simulink model "Old_control_speed"  (R2023b)
settings: Solver=ode1  StartTime=0.0  StopTime=inf  FixedStep=0.01  RelTol=1e-3
libraries: qbmove_library x3, simulink x2, QB_pacer_lib x1
settings Model: Creator=ilari  LastModifiedBy=ilari

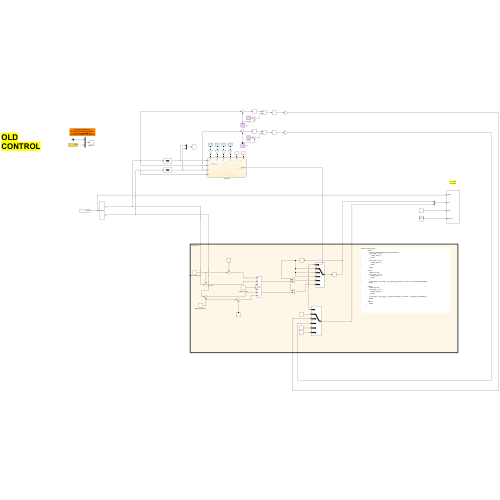
[thumbnail: Simulink's stored preview of the top-level diagram]
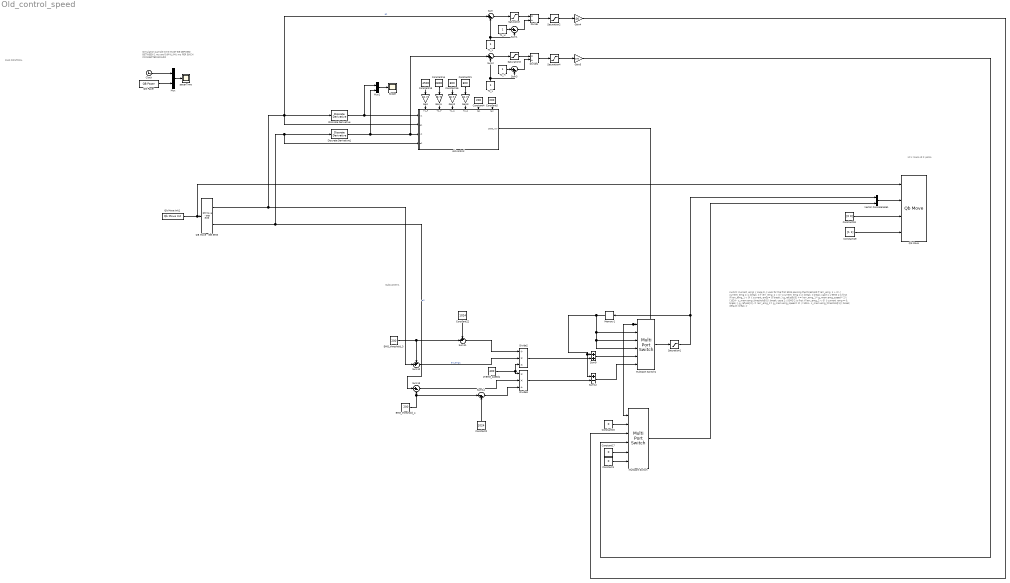
== system Old_control_speed ==
  note: Subsystem1
  note: OLD CONTROL
  note: id 1: mano
      | id 2: polso
  note: switch (current_emg) {
      | case 0:
      | // Look for the first EMG passing the threshold
      | if (err_emg_1 > 0) {
      | current_emg = 1;
      | break;
      | }
      | if (err_emg_2 > 0) {
      | current_emg = 2;
      | break;
      | }
      | break;
      |
      | case 1:
      | // EMG 1 is first
      | if (err_emg_1 < 0) {
      | current_emg = 0;
      | break;
      | }
      | g_ref.pos[0] += (err_emg_1 * g_mem.emg_speed * 2) / (1024 - c_mem.emg_threshold[0]);
      | break;
      |
      | case 2:
      | // EMG 2 is first
      | if (err_emg_2 < 0) {
      | current_emg = 0;
      | break;
      | }
      | g_ref.pos[0] -= (err_emg_2 * g_mem.emg_speed * 2) / (1024 - c_mem.emg_threshold[1]);
      | break;
      |
      | default:
      | break;
      | }
  note: Simulation sample time
      | MUST BE DEFINED BETWEEN
      | 1 ms and 0.6*N_IMU ms
      | PER EACH CONNECTED BOARD
  2*EMG_speed1 : Constant  Value=400
  Clock : Clock
  Constant1 : Constant  Value=0
  Constant13 : Constant  Value=4500
  Constant14 : Constant  Value=2800
  Constant15 : Constant  Value=0
  Constant16 : Constant  Value=800
  Constant17 : Constant  Value=0
  Constant18 : Constant  Value=[0 0]
  Constant19 : Constant  Value=[1 1]
  Constant2 : Constant  Value=1024
  Constant21 : Constant  Value=800
  Constant22 : Constant  Value=1024
  Constant4 : Constant  Value=200
  Constant5 : Constant  Value=200
  Discrete Derivative : simulink/Discrete/Discrete Derivative  gainval=1.0  ICPrevScaledInput=0.0  OutMin=[]  OutMax=[]  OutDataType=fixdt(1, 16)  OutScaling=2^-10  DoSatur=off
  Discrete Derivative1 : simulink/Discrete/Discrete Derivative  gainval=1.0  ICPrevScaledInput=0.0  OutMin=[]  OutMax=[]  OutDataType=fixdt(1, 16)  OutScaling=2^-10  DoSatur=off
  Divide : Product  Inputs=*/
  Divide1 : Product  Inputs=*/
  Divide2 : Product  Inputs=/**
  Divide3 : Product  Inputs=**/
  EMG_threshold_3 : Constant  Value=200
  EMG_threshold_4 : Constant  Value=200
  Gain{,1..3} (4 alike) : Gain  Gain=0.7
  Gain4 : Gain  Gain=100
  Gain5 : Gain  Gain=-100
  Memory1 : Memory
  Multiport Switch : MultiPortSwitch  DataPortOrder=Zero-based contiguous  Inputs=5  zeroidx=on  SaturateOnIntegerOverflow=off  InputSameDT=off
  Multiport Switch1 : MultiPortSwitch  DataPortOrder=Zero-based contiguous  Inputs=5  zeroidx=on  SaturateOnIntegerOverflow=off  InputSameDT=off
  Mux : Mux  Inputs=2
  Mux1 : Mux  Inputs=2
  QB Move - Get EMG : qbmove_library/QB Move - Get EMG  ID=2  DAISY_CHAINING=off
      settings: SourceProductName=Qb Move Library
  QB Pacer : QB_pacer_lib/QB Pacer  simTimePerRealTime=1
      settings: SourceProductName=QB Pacer
  Qb Move : qbmove_library/Qb Move  ID=[1 2]  ACTIVE_COMM_DIRECTIONS=Tx  CONTROL_MODE=Prime Movers Positions  DAISY_CHAINING=off  MAX_ANG=0  SW_LIMIT=inf  OFFSET=0  ACTIVATE=off  WDT=0.0  UNIT=TICK
      settings: LibrarySourceBlock=qbmove_library/qbmove  SourceProductName=Qb Move Library
  Qb Move Init1 : qbmove_library/Qb Move Init  NUMBER_OF_COM='COM9'  BAUD_RATE_COM=2000000
      settings: SourceProductName=Qb Move Library
  Saturation : Saturate  UpperLimit=inf  LowerLimit=0
  Saturation1 : Saturate  UpperLimit=17500  LowerLimit=0
  Saturation2 : Saturate  UpperLimit=1  LowerLimit=0.2
  Saturation3 : Saturate  UpperLimit=inf  LowerLimit=0
  Saturation4 : Saturate  UpperLimit=1  LowerLimit=0.45
  Scope : Scope
  Sum{,1..3,13} (5 alike) : Sum  Inputs=|+-
  Sum10 : Sum  Inputs=-+|
  Sum11 : Sum  Inputs=+-|
  Sum12 : Sum  Inputs=+-
  Sum14 : Sum  Inputs=|-+
  Sum9 : Sum
  T1_H : Constant
  T1_L : Constant
  T2_H : Constant
  T2_L : Constant
  Vector Concatenate1 : Concatenate
  old control : Stateflow chart  TreatAsAtomicUnit=on
      settings: PortSchema="{\"entries\":[{\"content\":{\"sides\":[{\"content\":{\"connectorIds\":[\"In9\",\"In2\",\"In10\",\"In3\"]},\"type\":\"ConnectorPlacement.EquallySpacedRectSide\",\"uuid\":\"aaa81814-6111-40a9-8a49-70dedea376f8\"},{\"content\":{\"connectorIds\":[\"Out1\"],\"side\":\"RIGHT\"},\"type\":\"ConnectorPlacement.EquallySpacedRectSide\",\"uuid\":\"4f5d7e2f-474c-41be-9ef6-4ca0a99bad8f\"},{\"content\":{\"connectorIds\":[\"In1\",\"In4\",\"In5\",\"In6\",\"In7\",\"In8\"],\"side\":\"TOP\"},\"type\":\"ConnectorPlacement.EquallySpacedRectSide\",\"uuid\":\"331e9dcb-f1b0-4631-9fd0-5bd3f1c908c0\"}]},\"type\":\"ConnectorPlacement.EquallySpacedConnector\",\"uuid\":\"41772918-0ee4-4ce1-8105-a12f23df084d\"}],\"packageUris\":[\"http://schema.mathworks.com/mf0/Connector/R2020b\"],\"version\":\"1.0\"}"
  pacerTime : Scope
  wires:
  Discrete Derivative1/1 -> Sum2/1, old control/10(v2), Mux1/2
  Discrete Derivative/1 -> old control/9(v1), Mux1/1
  Constant14/1 -> Gain1/1
  Constant19/1 -> Qb Move/4
  QB Move - Get EMG/1 -> Sum10/2, Sum/1, Discrete Derivative/1, old control/2(e1)  "e1"
  Constant13/1 -> Gain/1
  Vector Concatenate1/1 -> Qb Move/2
  QB Move - Get EMG/2 -> Sum13/1, Discrete Derivative1/1, old control/3(e2)  "e2"
  Constant18/1 -> Qb Move/3
  Qb Move Init1/1 -> Qb Move/1, QB Move - Get EMG/1
  Constant15/1 -> Multiport Switch/2
  Saturation1/1 -> Vector Concatenate1/1, Memory1/1
  Constant17/1 -> Multiport Switch/5
  Multiport Switch/1 -> Vector Concatenate1/2
  Constant22/1 -> Sum11/1
  Sum10/1 -> Divide2/2  "err_emg1"
  Sum13/1 -> Divide3/2
  2*EMG_speed1/1 -> Divide3/1, Divide2/3
  Constant2/1 -> Sum14/2
  EMG_threshold_4/1 -> Sum14/1, Sum13/2
  EMG_threshold_3/1 -> Sum10/1, Sum11/2
  Sum14/1 -> Divide3/3
  Divide3/1 -> Sum12/2
  Divide2/1 -> Sum9/2
  Sum11/1 -> Divide2/1
  Memory1/1 -> Multiport Switch1/3, Multiport Switch1/4, Multiport Switch1/2, Sum12/1, Sum9/1
  Multiport Switch1/1 -> Saturation1/1
  old control/1(state_var) -> Multiport Switch/1, Multiport Switch1/1
  Constant1/1 -> Multiport Switch/6
  Sum12/1 -> Multiport Switch1/6
  Sum9/1 -> Multiport Switch1/5
  Mux/1 -> pacerTime/1
  Clock/1 -> Mux/1
  QB Pacer/1 -> Mux/2
  Constant5/1 -> old control/8(te2)
  Constant4/1 -> old control/7(te1)
  Gain3/1 -> old control/6(T2_S)
  Gain2/1 -> old control/5(T1_S)
  Gain1/1 -> old control/4(T2_F)
  Gain/1 -> old control/1(T1_F)
  Sum/1 -> Saturation/1
  Saturation/1 -> Divide/1
  Sum1/1 -> Divide/2
  Divide/1 -> Saturation2/1
  Saturation2/1 -> Gain4/1
  Sum2/1 -> Saturation3/1
  Saturation3/1 -> Divide1/1
  Sum3/1 -> Divide1/2
  Saturation4/1 -> Gain5/1
  Divide1/1 -> Saturation4/1
  Constant21/1 -> Gain3/1
  Mux1/1 -> Scope/1
  Constant16/1 -> Gain2/1
  T1_L/1 -> Sum1/2, Sum/2
  T1_H/1 -> Sum1/1
  T2_H/1 -> Sum3/1
  T2_L/1 -> Sum3/2, Sum2/2
  Gain5/1 -> Multiport Switch/4
  Gain4/1 -> Multiport Switch/3

== stateflow chart Old_control_speed/old control ==
  state State1
    entry : state_var =1;
  note: WRIST ACTIVE - CLOCKWISE
  note: REST
  note: e1 (blu) veloce - chiude
      | e2 (nero) veloce - apre
      | e1 (blu) lento - rotazione oraria
      | e2 (nero) lento - rotazione antioraria
  state State3
    entry : state_var =3;
  state State0
    entry : state_var =0;
  note: CLOSE HAND
  state State2
    entry : state_var =2;
  note: WRIST ACTIVE - COUNTERCLOCKWISE
  note: OPEN HAND
  state State4
    entry : state_var =4;
  State0 -> State1 [order 1] : [v1<T1_F && v1>T1_S]
  State1 -> State0 : [e1<te1 ]
  State0 -> State3 [order 3] : [v1 > T1_F]
  State3 -> State0 : [e1<te1]
  (default) -> State0
  State4 -> State0 : [e2<te2]
  State0 -> State4 [order 4] : [v2>T2_F]
  State2 -> State0 : [e2 <te2 ]
  State0 -> State2 [order 2] : [v2<T2_F && v2>T2_S]
  data: T1_F input; e1 input; e2 input; T2_F input; T1_S input; T2_S input; te1 input; te2 input; v1 input; v2 input; state_var output
